simulink model "NMG_DMPC_Final"  (R2024b)
settings: Solver=VariableStepAuto  StartTime=0.0  StopTime=100  RelTol=1e-3
libraries: spspowerguiLib x1
settings Model: Creator=hp  LastModifiedBy=Ekko
settings SolverCC: AlgebraicLoopSolver=TrustRegion
settings DataIOCC: ReturnWorkspaceOutputs=off
settings DebuggingCC: UnconnectedInputMsg=warning  UnconnectedOutputMsg=warning  UnconnectedLineMsg=warning  ArithmeticOperatorsInVariantConditions=warning
settings ModelReferenceCC: EnableRefExpFcnMdlSchedulingChecks=on
settings SFSimCC: CustomCodeUndefinedFunction=UseInterfaceOnly
settings RTWCC: GPUComputeCapability=3.5

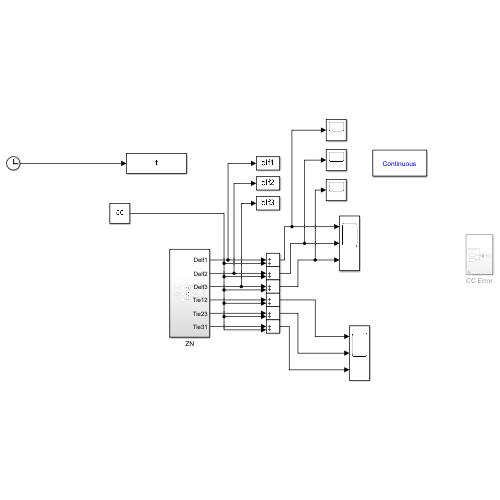
[thumbnail: Simulink's stored preview of the top-level diagram]
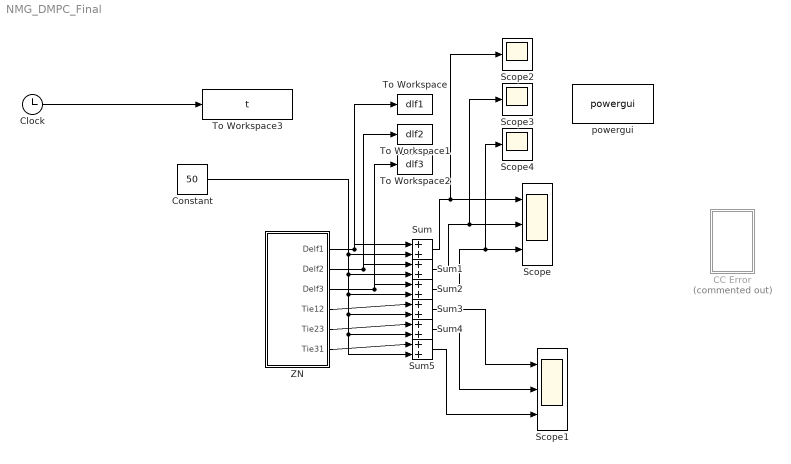
== system NMG_DMPC_Final ==
  CC Error : Subsystem  Commented=on
  Clock : Clock
  Constant : Constant  Value=50
  Scope : Scope  NumInputPorts=3
  Scope1 : Scope  NumInputPorts=3
  Scope2 : Scope
  Scope3 : Scope
  Scope4 : Scope
  Sum{,1..5} (6 alike) : Sum  Inputs=|++
  To Workspace : ToWorkspace  VariableName=dlf1  SampleTime=-1
      settings: Save2DSignal=2-D array (concatenate along first dimension)
  To Workspace1 : ToWorkspace  VariableName=dlf2  SampleTime=-1
      settings: Save2DSignal=2-D array (concatenate along first dimension)
  To Workspace2 : ToWorkspace  VariableName=dlf3  SampleTime=-1
      settings: Save2DSignal=2-D array (concatenate along first dimension)
  To Workspace3 : ToWorkspace  VariableName=t  SampleTime=-1
      settings: Save2DSignal=2-D array (concatenate along first dimension)
  ZN : Subsystem
  powergui : spspowerguiLib/powergui  Priority=1  SimulationMode=Continuous  SampleTime=50e-6  frequency=60  Iterations=50  frequencyindice=60  Pbase=100e6  ErrMax=1e-4  UnitsV=kV  UnitsW=MW  buscounter=0  FunctionMessages=off  echomessages=off  EnableUseOfTLC=off  CurrentSourceSwitches=off  DisableSnubberDevices=off  DisableRonSwitches=off  DisableVfSwitches=off  DisplayEquations=off  AutomaticDiscreteSolvers=off  SolverType=Tustin/Backward Euler (TBE)  Interpol=off  ExternalGateDelay=off  methode=off  Ts=100  x0status=blocks  SPID=on  SwTol=0  HookPort=off  NonlinearTolerance=1e-4  nMaxIteration=100  ContinueOnMaxIteration=off  RestoreLinks=warning  ResistiveCurrentMeasurement=off  Frange=[0:2:500]  Ylog=off  Xlog=on  ShowGrid=off  save=off  variable=ZData  structure=0  ZoomFFT=off  StartTime=0.0  cycles=1  DisplayStyle=1  fundamental=60  FreqAxis=off  MaxFrequency=1000  frequencyindicesteady=1  RmsSteady=1  display=off
  wires:
  ZN/1(Delf1) -> Sum/1, To Workspace/1
  Sum/1 -> Scope/1, Scope2/1
  Constant/1 -> Sum1/2, Sum3/2, Sum4/2, Sum5/2, Sum2/2, Sum/2
  ZN/2(Delf2) -> Sum1/1, To Workspace1/1
  ZN/3(Delf3) -> To Workspace2/1, Sum2/1
  Sum1/1 -> Scope3/1, Scope/2
  Sum2/1 -> Scope4/1, Scope/3
  ZN/4(Tie12) -> Sum3/1
  ZN/5(Tie23) -> Sum4/1
  ZN/6(Tie31) -> Sum5/1
  Sum3/1 -> Scope1/1
  Sum4/1 -> Scope1/2
  Sum5/1 -> Scope1/3
  Clock/1 -> To Workspace3/1

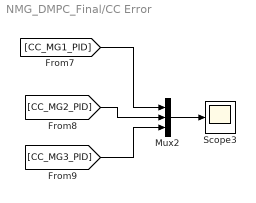
== system NMG_DMPC_Final/CC Error ==
  Mux2 : Mux  Inputs=3
  Scope3 : Scope
  wires:
  [CC_MG3_PID] -> Mux2/3
  Mux2/1 -> Scope3/1
  [CC_MG1_PID] -> Mux2/1
  [CC_MG2_PID] -> Mux2/2

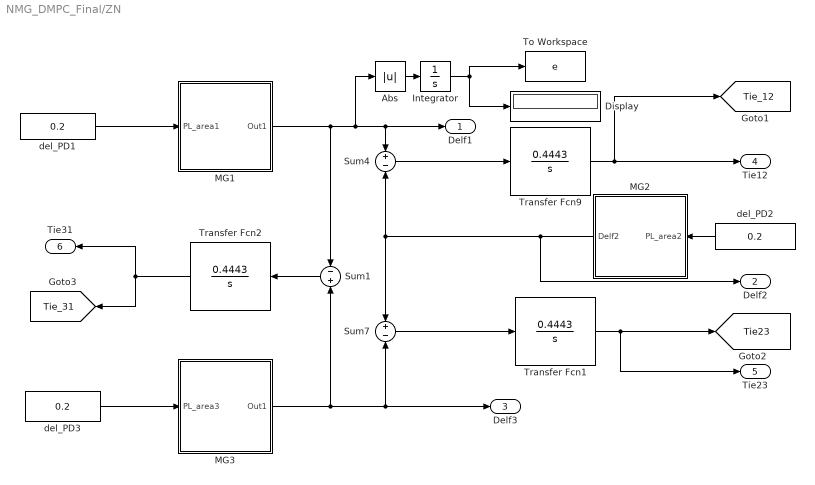
== system NMG_DMPC_Final/ZN ==
  Abs : Abs  SaturateOnIntegerOverflow=off
  Display : Display
  Integrator : Integrator
  MG1 : Subsystem
  MG2 : Subsystem
  MG3 : Subsystem
  Sum1 : Sum  Inputs=-+
  Sum4 : Sum  Inputs=+-
  Sum7 : Sum  Inputs=+-
  To Workspace : ToWorkspace  VariableName=e  SaveFormat=Timeseries  SampleTime=-1
  Transfer Fcn1 : TransferFcn  Numerator=[0.4443]  Denominator=[1 0]
  Transfer Fcn2 : TransferFcn  Numerator=[0.4443]  Denominator=[1 0]
  Transfer Fcn9 : TransferFcn  Numerator=[0.4443]  Denominator=[1 0]
  del_PD1 : Constant  Value=0.2
  del_PD2 : Constant  Value=0.2
  del_PD3 : Constant  Value=0.2
  Delf1 : Outport  VectorParamsAs1DForOutWhenUnconnected=off
  Delf2 : Outport  Port=2  VectorParamsAs1DForOutWhenUnconnected=off
  Delf3 : Outport  Port=3  VectorParamsAs1DForOutWhenUnconnected=off
  Tie12 : Outport  Port=4  VectorParamsAs1DForOutWhenUnconnected=off
  Tie23 : Outport  Port=5  VectorParamsAs1DForOutWhenUnconnected=off
  Tie31 : Outport  Port=6  VectorParamsAs1DForOutWhenUnconnected=off
  tag scope: Tie23=global, Tie_12=global, Tie_31=global
  wires:
  MG3/1(Out1) -> Delf3/1, Sum7/2, Sum1/2
  Sum7/1 -> Transfer Fcn1/1
  Sum4/1 -> Transfer Fcn9/1
  Transfer Fcn1/1 -> Tie23/1, [Tie23]
  Transfer Fcn9/1 -> [Tie_12], Tie12/1
  Sum1/1 -> Transfer Fcn2/1
  Transfer Fcn2/1 -> Tie31/1, [Tie_31]
  Integrator/1 -> Display/1, To Workspace/1
  MG1/1(Out1) -> Sum1/1, Abs/1, Sum4/1, Delf1/1
  Abs/1 -> Integrator/1
  del_PD2/1 -> MG2/1(PL_area2)
  del_PD3/1 -> MG3/1(PL_area3)
  del_PD1/1 -> MG1/1(PL_area1)
  MG2/1(Delf2) -> Sum7/1, Sum4/2, Delf2/1

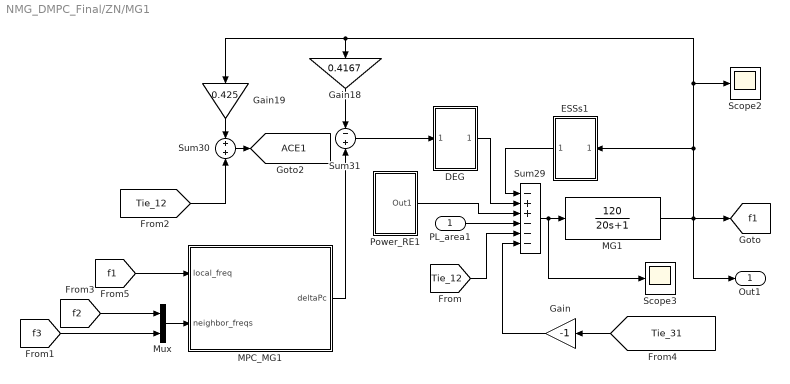
== system NMG_DMPC_Final/ZN/MG1 ==
  PL_area1 : Inport
  DEG : Subsystem
  ESSs1 : Subsystem
  Gain : Gain  Gain=-1
  Gain18 : Gain  Gain=0.4167
  Gain19 : Gain  Gain=0.425
  MG1 : TransferFcn  Numerator=[120]  Denominator=[20 1]
  MPC_MG1 : MATLAB Function  TreatAsAtomicUnit=on
  Mux : Mux  Inputs=2
  Power_RE1 : Subsystem
  Scope2 : Scope
  Scope3 : Scope
  Sum29 : Sum  Inputs=-++---
  Sum30 : Sum
  Sum31 : Sum  Inputs=-+
  Out1 : Outport  VectorParamsAs1DForOutWhenUnconnected=off
  tag scope: ACE1=global, f1=global
  wires:
  ESSs1/1(Out1) -> Sum29/1
  [Tie_12] -> Sum29/5
  MG1/1 -> [f1], Out1/1, ESSs1/1(In1), Scope2/1, Gain19/1, Gain18/1
  Sum29/1 -> Scope3/1, MG1/1
  Gain18/1 -> Sum31/1
  [Tie_12] -> Sum30/2
  MPC_MG1/1(deltaPc) -> Sum31/2
  Gain19/1 -> Sum30/1
  PL_area1/1 -> Sum29/4
  DEG/1(Out1) -> Sum29/2
  Power_RE1/1(Out1) -> Sum29/3
  Sum31/1 -> DEG/1(In1)
  [Tie_31] -> Gain/1
  Gain/1 -> Sum29/6
  Sum30/1 -> [ACE1]
  Mux/1 -> MPC_MG1/2(neighbor_freqs)
  [f2] -> Mux/1
  [f3] -> Mux/2
  [f1] -> MPC_MG1/1(local_freq)

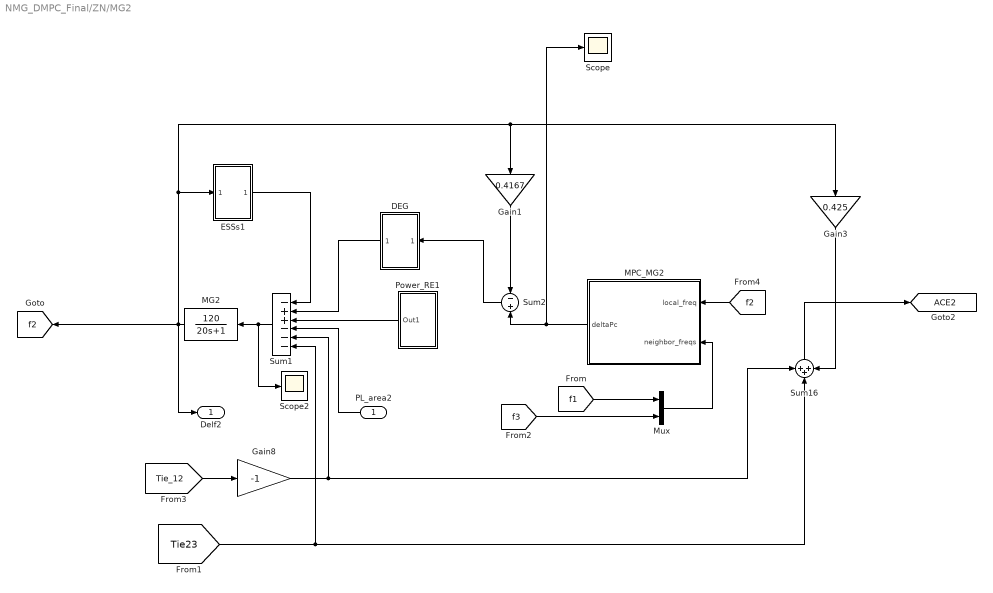
== system NMG_DMPC_Final/ZN/MG2 ==
  PL_area2 : Inport
  DEG : Subsystem
  ESSs1 : Subsystem
  Gain1 : Gain  Gain=0.4167
  Gain3 : Gain  Gain=0.425
  Gain8 : Gain  Gain=-1
  MG2 : TransferFcn  Numerator=[120]  Denominator=[20 1]
  MPC_MG2 : MATLAB Function  TreatAsAtomicUnit=on
  Mux : Mux  Inputs=2
  Power_RE1 : Subsystem
  Scope : Scope
  Scope2 : Scope
  Sum1 : Sum  Inputs=-++---
  Sum16 : Sum  Inputs=+++
  Sum2 : Sum  Inputs=-+
  Delf2 : Outport  VectorParamsAs1DForOutWhenUnconnected=off
  tag scope: ACE2=global, f2=global
  wires:
  [Tie23] -> Sum1/6, Sum16/2
  [Tie_12] -> Gain8/1
  MG2/1 -> ESSs1/1(In1), Gain1/1, Gain3/1, [f2], Delf2/1
  Gain8/1 -> Sum1/5, Sum16/1
  PL_area2/1 -> Sum1/4
  Gain1/1 -> Sum2/1
  MPC_MG2/1(deltaPc) -> Scope/1, Sum2/2
  Sum1/1 -> Scope2/1, MG2/1
  ESSs1/1(Out1) -> Sum1/1
  Gain3/1 -> Sum16/3
  DEG/1(Out1) -> Sum1/2
  Power_RE1/1(Out1) -> Sum1/3
  Sum2/1 -> DEG/1(In1)
  Sum16/1 -> [ACE2]
  Mux/1 -> MPC_MG2/2(neighbor_freqs)
  [f1] -> Mux/1
  [f3] -> Mux/2
  [f2] -> MPC_MG2/1(local_freq)

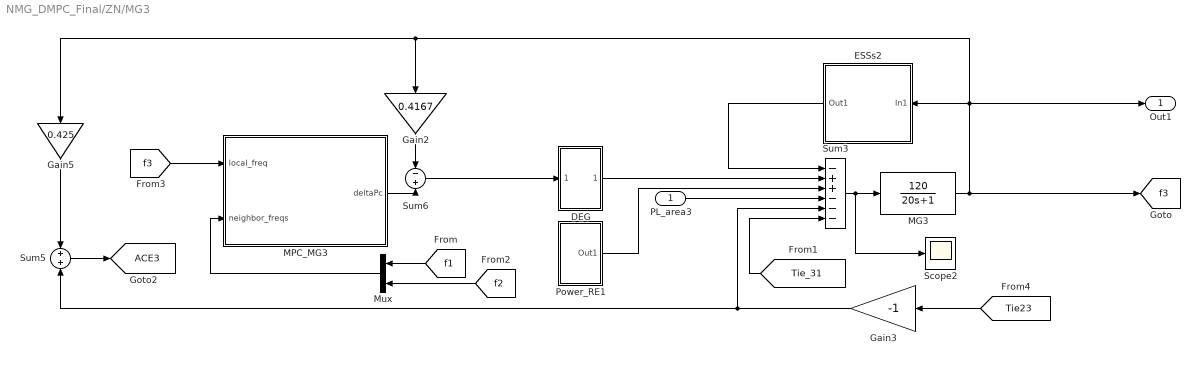
== system NMG_DMPC_Final/ZN/MG3 ==
  PL_area3 : Inport
  DEG : Subsystem
  ESSs2 : Subsystem
  Gain2 : Gain  Gain=0.4167
  Gain3 : Gain  Gain=-1
  Gain5 : Gain  Gain=0.425
  MG3 : TransferFcn  Numerator=[120]  Denominator=[20 1]
  MPC_MG3 : MATLAB Function  TreatAsAtomicUnit=on
  Mux : Mux  Inputs=2
  Power_RE1 : Subsystem
  Scope2 : Scope
  Sum3 : Sum  Inputs=-++---
  Sum5 : Sum
  Sum6 : Sum  Inputs=-+
  Out1 : Outport  VectorParamsAs1DForOutWhenUnconnected=off
  tag scope: ACE3=global, f3=global
  wires:
  MPC_MG3/1(deltaPc) -> Sum6/2
  Gain3/1 -> Sum3/5, Sum5/2
  MG3/1 -> [f3], Gain5/1, Gain2/1, Out1/1, ESSs2/1(In1)
  [Tie23] -> Gain3/1
  ESSs2/1(Out1) -> Sum3/1
  Gain2/1 -> Sum6/1
  Sum3/1 -> Scope2/1, MG3/1
  PL_area3/1 -> Sum3/4
  Power_RE1/1(Out1) -> Sum3/3
  Gain5/1 -> Sum5/1
  DEG/1(Out1) -> Sum3/2
  Sum6/1 -> DEG/1(In1)
  [Tie_31] -> Sum3/6
  Sum5/1 -> [ACE3]
  Mux/1 -> MPC_MG3/2(neighbor_freqs)
  [f2] -> Mux/2
  [f1] -> Mux/1
  [f3] -> MPC_MG3/1(local_freq)

== system NMG_DMPC_Final/ZN/MG1/DEG ==
  In1 : Inport
  Transfer Fcn15 : TransferFcn  Denominator=[1 1]
  Transfer Fcn22 : TransferFcn  Denominator=[2 1]
  Out1 : Outport  VectorParamsAs1DForOutWhenUnconnected=off
  wires:
  Transfer Fcn22/1 -> Transfer Fcn15/1
  In1/1 -> Transfer Fcn22/1
  Transfer Fcn15/1 -> Out1/1

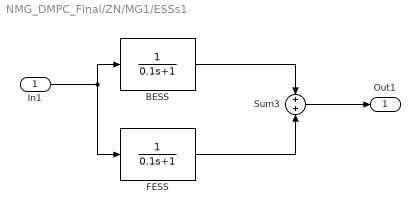
== system NMG_DMPC_Final/ZN/MG1/ESSs1 ==
  In1 : Inport
  BESS : TransferFcn  Denominator=[0.1 1]
  FESS : TransferFcn  Denominator=[0.1 1]
  Sum3 : Sum
  Out1 : Outport  VectorParamsAs1DForOutWhenUnconnected=off
  wires:
  In1/1 -> FESS/1, BESS/1
  Sum3/1 -> Out1/1
  FESS/1 -> Sum3/2
  BESS/1 -> Sum3/1

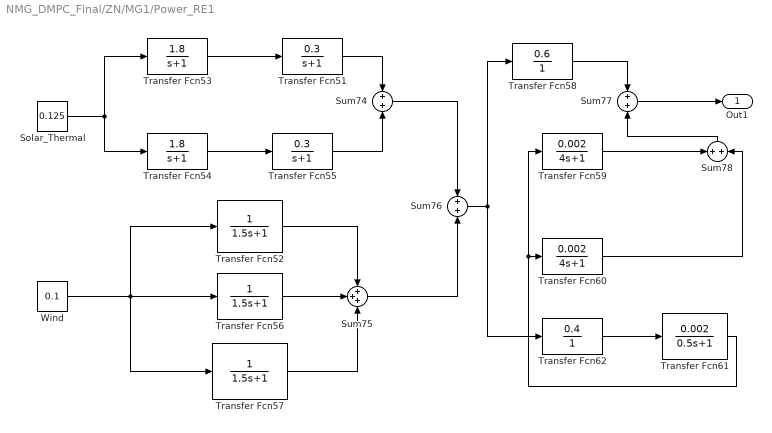
== system NMG_DMPC_Final/ZN/MG1/Power_RE1 ==
  Solar_Thermal : Constant  Value=0.125
  Sum{74,76..78} (4 alike) : Sum
  Sum75 : Sum  Inputs=+++
  Transfer Fcn51 : TransferFcn  Numerator=[0.3]  Denominator=[1 1]
  Transfer Fcn52 : TransferFcn  Denominator=[1.5 1]
  Transfer Fcn53 : TransferFcn  Numerator=[1.8]  Denominator=[1 1]
  Transfer Fcn54 : TransferFcn  Numerator=[1.8]  Denominator=[1 1]
  Transfer Fcn55 : TransferFcn  Numerator=[0.3]  Denominator=[1 1]
  Transfer Fcn56 : TransferFcn  Denominator=[1.5 1]
  Transfer Fcn57 : TransferFcn  Denominator=[1.5 1]
  Transfer Fcn58 : TransferFcn  Numerator=[0.6]  Denominator=[1]
  Transfer Fcn59 : TransferFcn  Numerator=[0.002]  Denominator=[4 1]
  Transfer Fcn60 : TransferFcn  Numerator=[0.002]  Denominator=[4 1]
  Transfer Fcn61 : TransferFcn  Numerator=[0.002]  Denominator=[0.5 1]
  Transfer Fcn62 : TransferFcn  Numerator=[0.4]  Denominator=[1]
  Wind : Constant  Value=0.1
  Out1 : Outport  VectorParamsAs1DForOutWhenUnconnected=off
  wires:
  Transfer Fcn52/1 -> Sum75/1
  Transfer Fcn53/1 -> Transfer Fcn51/1
  Solar_Thermal/1 -> Transfer Fcn53/1, Transfer Fcn54/1
  Transfer Fcn51/1 -> Sum74/1
  Transfer Fcn60/1 -> Sum78/2
  Transfer Fcn56/1 -> Sum75/2
  Wind/1 -> Transfer Fcn57/1, Transfer Fcn56/1, Transfer Fcn52/1
  Transfer Fcn57/1 -> Sum75/3
  Transfer Fcn58/1 -> Sum77/1
  Sum75/1 -> Sum76/2
  Sum78/1 -> Sum77/2
  Sum74/1 -> Sum76/1
  Transfer Fcn54/1 -> Transfer Fcn55/1
  Transfer Fcn55/1 -> Sum74/2
  Transfer Fcn61/1 -> Transfer Fcn60/1, Transfer Fcn59/1
  Transfer Fcn59/1 -> Sum78/1
  Sum76/1 -> Transfer Fcn58/1, Transfer Fcn62/1
  Transfer Fcn62/1 -> Transfer Fcn61/1
  Sum77/1 -> Out1/1

== system NMG_DMPC_Final/ZN/MG2/DEG ==
  In1 : Inport
  Transfer Fcn15 : TransferFcn  Denominator=[1 1]
  Transfer Fcn22 : TransferFcn  Denominator=[2 1]
  Out1 : Outport  VectorParamsAs1DForOutWhenUnconnected=off
  wires:
  Transfer Fcn22/1 -> Transfer Fcn15/1
  In1/1 -> Transfer Fcn22/1
  Transfer Fcn15/1 -> Out1/1

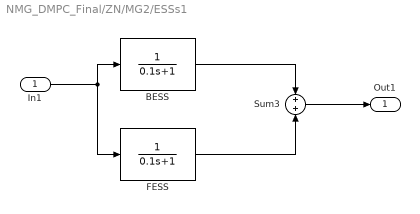
== system NMG_DMPC_Final/ZN/MG2/ESSs1 ==
  In1 : Inport
  BESS : TransferFcn  Denominator=[0.1 1]
  FESS : TransferFcn  Denominator=[0.1 1]
  Sum3 : Sum
  Out1 : Outport  VectorParamsAs1DForOutWhenUnconnected=off
  wires:
  In1/1 -> FESS/1, BESS/1
  Sum3/1 -> Out1/1
  FESS/1 -> Sum3/2
  BESS/1 -> Sum3/1

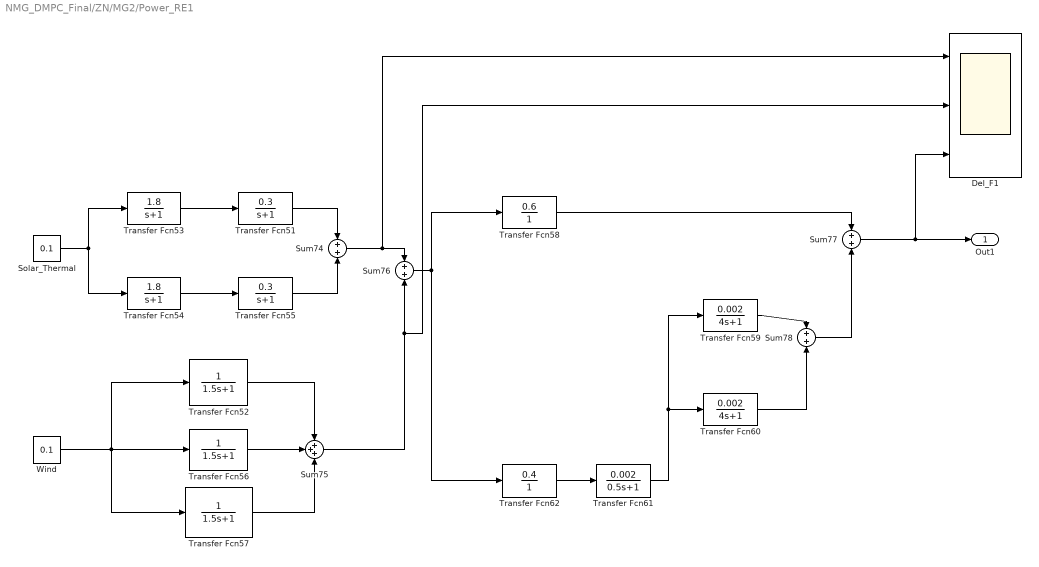
== system NMG_DMPC_Final/ZN/MG2/Power_RE1 ==
  Del_F1 : Scope  NumInputPorts=3
  Solar_Thermal : Constant  Value=0.1
  Sum{74,76..78} (4 alike) : Sum
  Sum75 : Sum  Inputs=+++
  Transfer Fcn51 : TransferFcn  Numerator=[0.3]  Denominator=[1 1]
  Transfer Fcn52 : TransferFcn  Denominator=[1.5 1]
  Transfer Fcn53 : TransferFcn  Numerator=[1.8]  Denominator=[1 1]
  Transfer Fcn54 : TransferFcn  Numerator=[1.8]  Denominator=[1 1]
  Transfer Fcn55 : TransferFcn  Numerator=[0.3]  Denominator=[1 1]
  Transfer Fcn56 : TransferFcn  Denominator=[1.5 1]
  Transfer Fcn57 : TransferFcn  Denominator=[1.5 1]
  Transfer Fcn58 : TransferFcn  Numerator=[0.6]  Denominator=[1]
  Transfer Fcn59 : TransferFcn  Numerator=[0.002]  Denominator=[4 1]
  Transfer Fcn60 : TransferFcn  Numerator=[0.002]  Denominator=[4 1]
  Transfer Fcn61 : TransferFcn  Numerator=[0.002]  Denominator=[0.5 1]
  Transfer Fcn62 : TransferFcn  Numerator=[0.4]  Denominator=[1]
  Wind : Constant  Value=0.1
  Out1 : Outport  VectorParamsAs1DForOutWhenUnconnected=off
  wires:
  Transfer Fcn52/1 -> Sum75/1
  Transfer Fcn53/1 -> Transfer Fcn51/1
  Solar_Thermal/1 -> Transfer Fcn54/1, Transfer Fcn53/1
  Transfer Fcn51/1 -> Sum74/1
  Transfer Fcn60/1 -> Sum78/2
  Transfer Fcn56/1 -> Sum75/2
  Wind/1 -> Transfer Fcn52/1, Transfer Fcn56/1, Transfer Fcn57/1
  Transfer Fcn57/1 -> Sum75/3
  Transfer Fcn58/1 -> Sum77/1
  Sum75/1 -> Del_F1/2, Sum76/2
  Sum78/1 -> Sum77/2
  Sum74/1 -> Del_F1/1, Sum76/1
  Transfer Fcn54/1 -> Transfer Fcn55/1
  Transfer Fcn55/1 -> Sum74/2
  Transfer Fcn61/1 -> Transfer Fcn60/1, Transfer Fcn59/1
  Transfer Fcn59/1 -> Sum78/1
  Sum76/1 -> Transfer Fcn62/1, Transfer Fcn58/1
  Transfer Fcn62/1 -> Transfer Fcn61/1
  Sum77/1 -> Del_F1/3, Out1/1

== system NMG_DMPC_Final/ZN/MG3/DEG ==
  In1 : Inport
  Transfer Fcn15 : TransferFcn  Denominator=[1 1]
  Transfer Fcn22 : TransferFcn  Denominator=[2 1]
  Out1 : Outport  VectorParamsAs1DForOutWhenUnconnected=off
  wires:
  Transfer Fcn22/1 -> Transfer Fcn15/1
  In1/1 -> Transfer Fcn22/1
  Transfer Fcn15/1 -> Out1/1

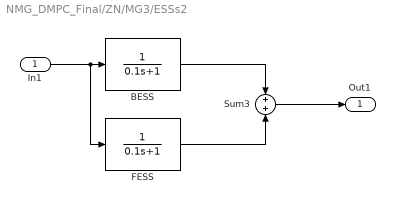
== system NMG_DMPC_Final/ZN/MG3/ESSs2 ==
  In1 : Inport
  BESS : TransferFcn  Denominator=[0.1 1]
  FESS : TransferFcn  Denominator=[0.1 1]
  Sum3 : Sum
  Out1 : Outport  VectorParamsAs1DForOutWhenUnconnected=off
  wires:
  BESS/1 -> Sum3/1
  FESS/1 -> Sum3/2
  In1/1 -> FESS/1, BESS/1
  Sum3/1 -> Out1/1

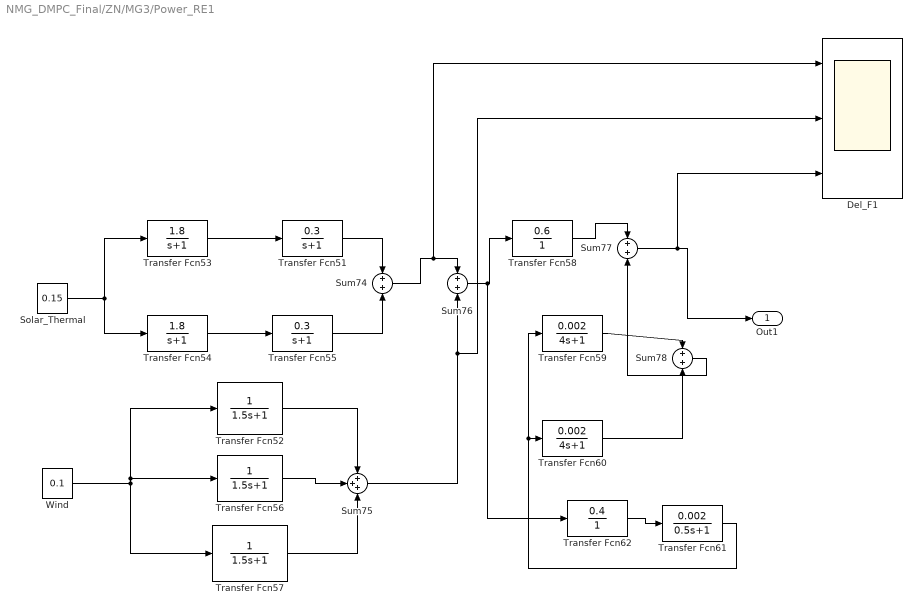
== system NMG_DMPC_Final/ZN/MG3/Power_RE1 ==
  Del_F1 : Scope  NumInputPorts=3
  Solar_Thermal : Constant  Value=0.15
  Sum{74,76..78} (4 alike) : Sum
  Sum75 : Sum  Inputs=+++
  Transfer Fcn51 : TransferFcn  Numerator=[0.3]  Denominator=[1 1]
  Transfer Fcn52 : TransferFcn  Denominator=[1.5 1]
  Transfer Fcn53 : TransferFcn  Numerator=[1.8]  Denominator=[1 1]
  Transfer Fcn54 : TransferFcn  Numerator=[1.8]  Denominator=[1 1]
  Transfer Fcn55 : TransferFcn  Numerator=[0.3]  Denominator=[1 1]
  Transfer Fcn56 : TransferFcn  Denominator=[1.5 1]
  Transfer Fcn57 : TransferFcn  Denominator=[1.5 1]
  Transfer Fcn58 : TransferFcn  Numerator=[0.6]  Denominator=[1]
  Transfer Fcn59 : TransferFcn  Numerator=[0.002]  Denominator=[4 1]
  Transfer Fcn60 : TransferFcn  Numerator=[0.002]  Denominator=[4 1]
  Transfer Fcn61 : TransferFcn  Numerator=[0.002]  Denominator=[0.5 1]
  Transfer Fcn62 : TransferFcn  Numerator=[0.4]  Denominator=[1]
  Wind : Constant  Value=0.1
  Out1 : Outport  VectorParamsAs1DForOutWhenUnconnected=off
  wires:
  Transfer Fcn52/1 -> Sum75/1
  Transfer Fcn53/1 -> Transfer Fcn51/1
  Solar_Thermal/1 -> Transfer Fcn53/1, Transfer Fcn54/1
  Transfer Fcn51/1 -> Sum74/1
  Transfer Fcn60/1 -> Sum78/2
  Transfer Fcn56/1 -> Sum75/2
  Wind/1 -> Transfer Fcn56/1, Transfer Fcn52/1, Transfer Fcn57/1
  Transfer Fcn57/1 -> Sum75/3
  Transfer Fcn58/1 -> Sum77/1
  Sum75/1 -> Del_F1/2, Sum76/2
  Sum78/1 -> Sum77/2
  Sum74/1 -> Del_F1/1, Sum76/1
  Transfer Fcn54/1 -> Transfer Fcn55/1
  Transfer Fcn55/1 -> Sum74/2
  Transfer Fcn61/1 -> Transfer Fcn60/1, Transfer Fcn59/1
  Transfer Fcn59/1 -> Sum78/1
  Sum76/1 -> Transfer Fcn62/1, Transfer Fcn58/1
  Transfer Fcn62/1 -> Transfer Fcn61/1
  Sum77/1 -> Del_F1/3, Out1/1

== matlab function NMG_DMPC_Final/ZN/MG1/MPC_MG1 ==
  settings: updateMethod=DISCRETE
  data: local_freq input; deltaPc output; neighbor_freqs input
function deltaPc = MPC_MG1(local_freq, neighbor_freqs)
    % System Parameters
    Ts = 0.01;          % Fixed sampling time (seconds)
    R_droop = 0.41667;  % Droop constant
    T12 = 0.4443;       % Tie-line coefficient MG1-MG2
    T31 = 0.4443;       % Tie-line coefficient MG3-MG1
    
    % MPC Design Parameters - Ultimate stability configuration
    Np = 20;        % Very long prediction horizon for maximum stability
    Nc = 5;         % Minimal control horizon for extremely smooth action
    
    % State-Space Matrices
    % States: [DEG(2) Solar(4) Wind(3) RE_Out(4) ESS(2) PS(3)]
    A = zeros(18, 18);  % Initialize with zeros for clarity
    
    % Fill in the A matrix blocks (keep your existing A matrix setup)
    % DEG dynamics (states 1-2)
    A(1:2, 1:2) = [-1/2, 0;
                    1,  -1];
    
    % Solar-Thermal (states 3-6)
    A(3:6, 3:6) = [-1,   1.8,   0,    0;
                    0,    -1,    0,    0;
                    0,     0,   -1,   0.3;
                    0,     0,    0,   -1];
                    
    % Wind (states 7-9)
    A(7:9, 7:9) = [-2/3,  0,    0;
                     0,   -2/3,  0;
                     0,    0,   -2/3];
                     
    % RE Output Stage (states 10-13)
    A(10, 3:9) = [1, 0, 1, 0, 1, 1, 1];  % Connections from Solar and Wind
    A(10:13, 10:13) = [-1/4,  0,    0,    0;
                        0,   -1/4,   0,    0;
                        0,    0.6,   0,    0;
                        0,     0,    0,   -2];
                        
    % ESS (states 14-15)
    A(14:15, 14:15) = [-10,  0;
                         0, -10];
                         
    % Power System & Tie-lines (states 16-18)
    A(16, [1,10:15]) = [120/20, 120/20, 120/20, 120/20, 120/20, 120/20, 120/20];  % Effects on frequency
    A(16:18, 16:18) = [-1/20,  0,    0;
                        T12,    0,    0;  % Tie-line to MG2
                        T31,    0,    0];  % Tie-line to MG3
    
    % Input matrix B
    B = zeros(18, 1);
    B(1) = 1/2;  % Control input only affects DEG first state
    
    % Output matrix C - only measure frequency for control
    C = zeros(1, 18);
    C(16) = 1;  % Measure frequency state
    
    % Augmented System
    A_aug = [A, zeros(18,1);
             C, 0];
    B_aug = [B; 0];
    C_aug = [C, 0];
    
    % Discrete-time conversion
    Ad = eye(19) + Ts*A_aug;
    Bd = Ts*B_aug;
    Cd = C_aug;
    
    % Persistent variables with enhanced filtering
    persistent x_est u_prev integral_error avg_error filter_count
    persistent y_hist error_trend deltaPc_hist prev_solution
    persistent y_filtered_prev deltaPc_final_prev
    if isempty(x_est)
        x_est = zeros(19, 1);
        u_prev = 0;
        integral_error = 0;
        avg_error = 0;
        filter_count = 0;
        y_hist = zeros(8, 1);
        error_trend = zeros(5, 1);
        deltaPc_hist = zeros(3, 1);
        prev_solution = zeros(Nc, 1);
        y_filtered_prev = 0;
        deltaPc_final_prev = 0;
    end
    
    % Extract frequency information from neighbors
    freq_MG2 = neighbor_freqs(1);
    freq_MG3 = neighbor_freqs(2);
    
    % Distributed Control Based on Laplacian Matrix
    % For MG1 (Leader): Use direct reference tracking + neighboring information
    reference = 50.0;  % Reference frequency
    graph_gain = 0.2;  % Gain for graph-based control
    
    % Calculate distributed control error using graph theory
    % Based on local error + weighted neighbor errors
    laplacian_error = 2*local_freq - freq_MG2 - freq_MG3;
    reference_error = local_freq - reference;
    
    % Combined error (leader node has direct access to reference)
    dist_error = reference_error + graph_gain*laplacian_error;
    
    % Enhanced measurement filtering with longer history and stronger filtering
    y_hist = [dist_error; y_hist(1:end-1)];
    
    % Two-stage filtering for maximum noise rejection
    % First stage: weighted moving average
    weights = [0.25, 0.2, 0.15, 0.1, 0.1, 0.08, 0.07, 0.05];
    weights = weights(1:min(length(weights), length(y_hist)));
    weights = weights / sum(weights);
    y_filtered_stage1 = y_hist' * weights';
    
    % Second stage: low-pass filter
    if isempty(y_filtered_prev)
        y_filtered_prev = y_filtered_stage1;
    end
    y_filtered = 0.8*y_filtered_prev + 0.2*y_filtered_stage1;
    y_filtered_prev = y_filtered;
    
    % Ultra-conservative integral action with wider dead zone
    error_signal = y_filtered;
    
    % Expanded dead zone with extremely slow integration
    if abs(error_signal) > 0.01
        integral_error = 0.99*integral_error + 0.01*Ts*error_signal*0.05;
    else
        % Inside dead zone - practically frozen integration
        integral_error = 0.9995*integral_error + 0.0005*Ts*error_signal*0.01;
    end
    
    % Moving average error for steady-state offset detection
    avg_error = 0.95*avg_error + 0.05*error_signal;
    filter_count = filter_count + 1;
    
    % State estimation with improved observer gain
    y_meas = y_filtered;
    x_est = Ad*x_est + Bd*u_prev;
    
    % Slightly increased observer gain for better tracking
    L = [0.08*ones(18,1); 0.12];
    x_est = x_est + L*(y_meas - Cd*x_est);
    x_est(19) = integral_error;
    
    % Prediction matrices
    [F, Phi] = getPredictionMatrices(Ad, Bd, Cd, Np, Nc);
    
    % Cost function weights - Critically over-damped response design
    % Extremely flat weight distribution for maximum smoothness
    %q_weights = exp(linspace(0, 0.2, Np));  % Very gradual weight increase
    Q = diag(500 * exp(linspace(0, 0.5, Np)));  % Sharper tracking
    
    % Ultra-high penalty on control moves to eliminate any oscillatory behavior
    R = diag(0.8 * ones(Nc,1));                 % Reduced control penalty
    
    % Reference trajectory - Targeting zero error
    r = zeros(Np,1);
    
    % Constraints - Extremely tight rate constraints for absolute stability
    du_max = 0.01;      % Minimal rate of change allowed
    u_max = 0.13;
    u_min = -0.13;
    
    % QP matrices
    [H, f] = getQPMatrices(F, Phi, Q, R, r, x_est);
    [A_ineq, b_ineq] = getConstraintMatrices(Nc, u_max, u_min, du_max, u_prev);
    
    % Initial guess - Use previous solution as starting point if available
    x0 = prev_solution;
    
    % Solve QP problem with improved options
    options = optimoptions('quadprog', 'Display', 'off', 'Algorithm', 'active-set', ...
                          'MaxIterations', 100);
    du = quadprog(H, f, A_ineq, b_ineq, [], [], [], [], x0, options);
    
    % Store solution for next iteration
    if ~isempty(du)
        prev_solution = du;
        delta_u = du(1);
    else
        delta_u = 0;
    end
    
    % Add anti-windup to prevent integral windup
    if abs(u_prev) >= u_max - 0.01
        integral_error = 0.9 * integral_error; % Reduce integral action when near constraints
    end
    
    % Maximum damping factor with triple-stage filtering
    % First stage - exponential smoothing with heavy bias toward previous value
    deltaPc_stage1 = 0.85*u_prev + 0.15*delta_u;
    
    % Second stage - moving average filter
    deltaPc_hist = [deltaPc_stage1; deltaPc_hist(1:end-1)];
    if all(deltaPc_hist == 0)
        deltaPc_hist = zeros(3, 1) + deltaPc_stage1;
    end
    deltaPc_stage2 = 0.7*deltaPc_hist(1) + 0.2*deltaPc_hist(2) + 0.1*deltaPc_hist(3);
    
    % Third stage - additional low-pass filter
    if isempty(deltaPc_final_prev)
        deltaPc_final_prev = deltaPc_stage2;
    end
    deltaPc = 0.9*deltaPc_final_prev + 0.1*deltaPc_stage2;
    deltaPc_final_prev = deltaPc;
    
    % Update persistent variables
    u_prev = deltaPc;
    
    return;
end

function [F, Phi] = getPredictionMatrices(A, B, C, Np, Nc)
    % Keep your existing function implementation
    [ny, nx] = size(C);
    F = zeros(Np, nx);
    Phi = zeros(Np, Nc);
    
    % Build F matrix
    for i = 1:Np
        F(i,:) = C * A^i;
    end
    
    % Build Phi matrix
    for i = 1:Np
        for j = 1:min(i,Nc)
            if i == j
                Phi(i,j) = C * B;
            else
                Phi(i,j) = C * A^(i-j) * B;
            end
        end
    end
end

function [H, f] = getQPMatrices(F, Phi, Q, R, r, x)
    % Keep your existing function implementation
    H = 2*(Phi'*Q*Phi + R);
    f = 2*Phi'*Q*(F*x - r);
end

function [A_ineq, b_ineq] = getConstraintMatrices(Nc, u_max, u_min, du_max, u_prev)
    % Keep your existing function implementation
    A_rate = [eye(Nc); -eye(Nc)];
    b_rate = [du_max*ones(Nc,1); du_max*ones(Nc,1)];
    
    A_input = tril(ones(Nc));
    A_amp = [A_input; -A_input];
    b_amp = [(u_max - u_prev)*ones(Nc,1); -(u_min - u_prev)*ones(Nc,1)];
    
    A_ineq = [A_rate; A_amp];
    b_ineq = [b_rate; b_amp];
end

== matlab function NMG_DMPC_Final/ZN/MG3/MPC_MG3 ==
  settings: updateMethod=DISCRETE
  data: local_freq input; deltaPc output; neighbor_freqs input
function deltaPc = MPC_MG3(local_freq, neighbor_freqs)
    % System Parameters
    Ts = 0.01;          % Fixed sampling time (seconds)
    R_droop = 0.41667;  % Droop constant
    T31 = 0.4443;       % Tie-line coefficient MG3-MG1
    T23 = 0.4443;       % Tie-line coefficient MG2-MG3
    
    % MPC Design Parameters - Ultimate stability configuration
    Np = 20;        % Very long prediction horizon for maximum stability
    Nc = 5;         % Minimal control horizon for extremely smooth action
    
    % State-Space Matrices
    % Keep your existing A matrix setup
    A = zeros(18, 18);  % Initialize with zeros for clarity
    
    % Fill in the A matrix blocks
    % DEG dynamics (states 1-2)
    A(1:2, 1:2) = [-1/2, 0;
                    1,  -1];
    
    % Solar-Thermal (states 3-6)
    A(3:6, 3:6) = [-1,   1.8,   0,    0;
                    0,    -1,    0,    0;
                    0,     0,   -1,   0.3;
                    0,     0,    0,   -1];
                    
    % Wind (states 7-9)
    A(7:9, 7:9) = [-2/3,  0,    0;
                     0,   -2/3,  0;
                     0,    0,   -2/3];
                     
    % RE Output Stage (states 10-13)
    A(10, 3:9) = [1, 0, 1, 0, 1, 1, 1];  % Connections from Solar and Wind
    A(10:13, 10:13) = [-1/4,  0,    0,    0;
                        0,   -1/4,   0,    0;
                        0,    0.6,   0,    0;
                        0,     0,    0,   -2];
                        
    % ESS (states 14-15)
    A(14:15, 14:15) = [-10,  0;
                         0, -10];
                         
    % Power System & Tie-lines (states 16-18)
    A(16, [1,10:15]) = [120/20, 120/20, 120/20, 120/20, 120/20, 120/20, 120/20];  % Effects on frequency
    A(16:18, 16:18) = [-1/20,  0,    0;
                        T31,    0,    0;  % Tie-line to MG1
                        T23,    0,    0];  % Tie-line to MG2
    
    % Input matrix B
    B = zeros(18, 1);
    B(1) = 1/2;  % Control input only affects DEG first state
    
    % Output matrix C - only measure frequency for control
    C = zeros(1, 18);
    C(16) = 1;  % Measure frequency state
    
    % Augmented System
    A_aug = [A, zeros(18,1);
             C, 0];
    B_aug = [B; 0];
    C_aug = [C, 0];
    
    % Discrete-time conversion
    Ad = eye(19) + Ts*A_aug;
    Bd = Ts*B_aug;
    Cd = C_aug;
    
    % Persistent variables with enhanced filtering
    persistent x_est u_prev integral_error avg_error filter_count
    persistent y_hist error_trend deltaPc_hist prev_solution
    persistent y_filtered_prev deltaPc_final_prev
    if isempty(x_est)
        x_est = zeros(19, 1);
        u_prev = 0;
        integral_error = 0;
        avg_error = 0;
        filter_count = 0;
        y_hist = zeros(8, 1);
        error_trend = zeros(5, 1);
        deltaPc_hist = zeros(3, 1);
        prev_solution = zeros(Nc, 1);
        y_filtered_prev = 0;
        deltaPc_final_prev = 0;
    end
    
    % Extract frequency information from neighbors
    freq_MG1 = neighbor_freqs(1);  % Leader frequency
    freq_MG2 = neighbor_freqs(2);
    
    % Distributed Control Based on Laplacian Matrix
    % For MG3 (Follower): Use neighboring information
    graph_gain = 0.2;  % Gain for graph-based control
    leader_gain = 0.5; % Higher gain for tracking the leader
    
    % Calculate distributed control error using graph theory
    % Based on local error + weighted neighbor errors
    laplacian_error = 2*local_freq - freq_MG1 - freq_MG2;
    leader_error = local_freq - freq_MG1;  % Track the leader
    
    % Combined error (follower node emphasizes tracking the leader)
    dist_error = leader_gain*leader_error + graph_gain*laplacian_error;
    
    % Enhanced measurement filtering with longer history and stronger filtering
    y_hist = [dist_error; y_hist(1:end-1)];
    
    % Two-stage filtering for maximum noise rejection
    % First stage: weighted moving average
    weights = [0.25, 0.2, 0.15, 0.1, 0.1, 0.08, 0.07, 0.05];
    weights = weights(1:min(length(weights), length(y_hist)));
    weights = weights / sum(weights);
    y_filtered_stage1 = y_hist' * weights';
    
    % Second stage: low-pass filter
    if isempty(y_filtered_prev)
        y_filtered_prev = y_filtered_stage1;
    end
    y_filtered = 0.8*y_filtered_prev + 0.2*y_filtered_stage1;
    y_filtered_prev = y_filtered;
    
    % Ultra-conservative integral action with wider dead zone
    error_signal = y_filtered;
    
    % Expanded dead zone with extremely slow integration
    if abs(error_signal) > 0.01
        integral_error = 0.99*integral_error + 0.01*Ts*error_signal*0.05;
    else
        % Inside dead zone - practically frozen integration
        integral_error = 0.9995*integral_error + 0.0005*Ts*error_signal*0.01;
    end
    
    % Moving average error for steady-state offset detection
    avg_error = 0.95*avg_error + 0.05*error_signal;
    filter_count = filter_count + 1;
    
    % State estimation with improved observer gain
    y_meas = y_filtered;
    x_est = Ad*x_est + Bd*u_prev;
    
    % Slightly increased observer gain for better tracking
    L = [0.08*ones(18,1); 0.12];
    x_est = x_est + L*(y_meas - Cd*x_est);
    x_est(19) = integral_error;
    
    % Prediction matrices
    [F, Phi] = getPredictionMatrices(Ad, Bd, Cd, Np, Nc);
    
    % Cost function weights - Critically over-damped response design
    % Extremely flat weight distribution for maximum smoothness
    %q_weights = exp(linspace(0, 0.2, Np));  % Very gradual weight increase
    Q = diag(500 * exp(linspace(0, 0.5, Np)));  % Sharper tracking
    
    % Ultra-high penalty on control moves to eliminate any oscillatory behavior
    R = diag(0.8 * ones(Nc,1));                 % Reduced control penalty
    
    % Reference trajectory - Targeting zero error
    r = zeros(Np,1);
    
    % Constraints - Extremely tight rate constraints for absolute stability
    du_max = 0.01;      % Minimal rate of change allowed
    u_max = 0.13;
    u_min = -0.13;
    % QP matrices
    [H, f] = getQPMatrices(F, Phi, Q, R, r, x_est);
    [A_ineq, b_ineq] = getConstraintMatrices(Nc, u_max, u_min, du_max, u_prev);
    
    % Initial guess - Use previous solution as starting point if available
    x0 = prev_solution;
    
    % Solve QP problem with improved options
    options = optimoptions('quadprog', 'Display', 'off', 'Algorithm', 'active-set', ...
                          'MaxIterations', 100);
    du = quadprog(H, f, A_ineq, b_ineq, [], [], [], [], x0, options);
    
    % Store solution for next iteration
    if ~isempty(du)
        prev_solution = du;
        delta_u = du(1);
    else
        delta_u = 0;
    end
    
    % Add anti-windup to prevent integral windup
    if abs(u_prev) >= u_max - 0.01
        integral_error = 0.9 * integral_error; % Reduce integral action when near constraints
    end
    
    % Maximum damping factor with triple-stage filtering
    % First stage - exponential smoothing with heavy bias toward previous value
    deltaPc_stage1 = 0.85*u_prev + 0.15*delta_u;
    
    % Second stage - moving average filter
    deltaPc_hist = [deltaPc_stage1; deltaPc_hist(1:end-1)];
    if all(deltaPc_hist == 0)
        deltaPc_hist = zeros(3, 1) + deltaPc_stage1;
    end
    deltaPc_stage2 = 0.7*deltaPc_hist(1) + 0.2*deltaPc_hist(2) + 0.1*deltaPc_hist(3);
    
    % Third stage - additional low-pass filter
    if isempty(deltaPc_final_prev)
        deltaPc_final_prev = deltaPc_stage2;
    end
    deltaPc = 0.9*deltaPc_final_prev + 0.1*deltaPc_stage2;
    deltaPc_final_prev = deltaPc;
    
    % Update persistent variables
    u_prev = deltaPc;
    
    return;
end

function [F, Phi] = getPredictionMatrices(A, B, C, Np, Nc)
    % Keep your existing function implementation
    [ny, nx] = size(C);
    F = zeros(Np, nx);
    Phi = zeros(Np, Nc);
    
    % Build F matrix
    for i = 1:Np
        F(i,:) = C * A^i;
    end
    
    % Build Phi matrix
    for i = 1:Np
        for j = 1:min(i,Nc)
            if i == j
                Phi(i,j) = C * B;
            else
                Phi(i,j) = C * A^(i-j) * B;
            end
        end
    end
end

function [H, f] = getQPMatrices(F, Phi, Q, R, r, x)
    % Keep your existing function implementation
    H = 2*(Phi'*Q*Phi + R);
    f = 2*Phi'*Q*(F*x - r);
end

function [A_ineq, b_ineq] = getConstraintMatrices(Nc, u_max, u_min, du_max, u_prev)
    % Keep your existing function implementation
    A_rate = [eye(Nc); -eye(Nc)];
    b_rate = [du_max*ones(Nc,1); du_max*ones(Nc,1)];
    
    A_input = tril(ones(Nc));
    A_amp = [A_input; -A_input];
    b_amp = [(u_max - u_prev)*ones(Nc,1); -(u_min - u_prev)*ones(Nc,1)];
    
    A_ineq = [A_rate; A_amp];
    b_ineq = [b_rate; b_amp];
end

== matlab function NMG_DMPC_Final/ZN/MG2/MPC_MG2 ==
  settings: updateMethod=DISCRETE
  data: local_freq input; deltaPc output; neighbor_freqs input
function deltaPc = MPC_MG2(local_freq, neighbor_freqs)
    % System Parameters
    Ts = 0.01;          % Fixed sampling time (seconds)
    R_droop = 0.41667;  % Droop constant
    T12 = 0.4443;       % Tie-line coefficient MG1-MG2
    T23 = 0.4443;       % Tie-line coefficient MG2-MG3
    
    % MPC Design Parameters - Ultimate stability configuration
    Np = 20;        % Very long prediction horizon for maximum stability
    Nc = 5;         % Minimal control horizon for extremely smooth action
    
    % State-Space Matrices
    % Keep your existing A matrix setup
    A = zeros(18, 18);  % Initialize with zeros for clarity
    
    % Fill in the A matrix blocks
    % DEG dynamics (states 1-2)
    A(1:2, 1:2) = [-1/2, 0;
                    1,  -1];
    
    % Solar-Thermal (states 3-6)
    A(3:6, 3:6) = [-1,   1.8,   0,    0;
                    0,    -1,    0,    0;
                    0,     0,   -1,   0.3;
                    0,     0,    0,   -1];
                    
    % Wind (states 7-9)
    A(7:9, 7:9) = [-2/3,  0,    0;
                     0,   -2/3,  0;
                     0,    0,   -2/3];
                     
    % RE Output Stage (states 10-13)
    A(10, 3:9) = [1, 0, 1, 0, 1, 1, 1];  % Connections from Solar and Wind
    A(10:13, 10:13) = [-1/4,  0,    0,    0;
                        0,   -1/4,   0,    0;
                        0,    0.6,   0,    0;
                        0,     0,    0,   -2];
                        
    % ESS (states 14-15)
    A(14:15, 14:15) = [-10,  0;
                         0, -10];
                         
    % Power System & Tie-lines (states 16-18)
    A(16, [1,10:15]) = [120/20, 120/20, 120/20, 120/20, 120/20, 120/20, 120/20];  % Effects on frequency
    A(16:18, 16:18) = [-1/20,  0,    0;
                        T12,    0,    0;  % Tie-line to MG1
                        T23,    0,    0];  % Tie-line to MG3
    
    % Input matrix B
    B = zeros(18, 1);
    B(1) = 1/2;  % Control input only affects DEG first state
    
    % Output matrix C - only measure frequency for control
    C = zeros(1, 18);
    C(16) = 1;  % Measure frequency state
    
    % Augmented System
    A_aug = [A, zeros(18,1);
             C, 0];
    B_aug = [B; 0];
    C_aug = [C, 0];
    
    % Discrete-time conversion
    Ad = eye(19) + Ts*A_aug;
    Bd = Ts*B_aug;
    Cd = C_aug;
    
    % Persistent variables with enhanced filtering
    persistent x_est u_prev integral_error avg_error filter_count
    persistent y_hist error_trend deltaPc_hist prev_solution
    persistent y_filtered_prev deltaPc_final_prev
    if isempty(x_est)
        x_est = zeros(19, 1);
        u_prev = 0;
        integral_error = 0;
        avg_error = 0;
        filter_count = 0;
        y_hist = zeros(8, 1);
        error_trend = zeros(5, 1);
        deltaPc_hist = zeros(3, 1);
        prev_solution = zeros(Nc, 1);
        y_filtered_prev = 0;
        deltaPc_final_prev = 0;
    end
    
    % Extract frequency information from neighbors
    freq_MG1 = neighbor_freqs(1);  % Leader frequency
    freq_MG3 = neighbor_freqs(2);
    
    % Distributed Control Based on Laplacian Matrix
    % For MG2 (Follower): Use neighboring information
    graph_gain = 0.2;  % Gain for graph-based control
    leader_gain = 0.5; % Higher gain for tracking the leader
    
    % Calculate distributed control error using graph theory
    % Based on local error + weighted neighbor errors
    laplacian_error = 2*local_freq - freq_MG1 - freq_MG3;
    leader_error = local_freq - freq_MG1;  % Track the leader
    
    % Combined error (follower node emphasizes tracking the leader)
    dist_error = leader_gain*leader_error + graph_gain*laplacian_error;
    
    % Enhanced measurement filtering with longer history and stronger filtering
    y_hist = [dist_error; y_hist(1:end-1)];
    
    % Two-stage filtering for maximum noise rejection
    % First stage: weighted moving average
    weights = [0.25, 0.2, 0.15, 0.1, 0.1, 0.08, 0.07, 0.05];
    weights = weights(1:min(length(weights), length(y_hist)));
    weights = weights / sum(weights);
    y_filtered_stage1 = y_hist' * weights';
    
    % Second stage: low-pass filter
    if isempty(y_filtered_prev)
        y_filtered_prev = y_filtered_stage1;
    end
    y_filtered = 0.8*y_filtered_prev + 0.2*y_filtered_stage1;
    y_filtered_prev = y_filtered;
    
    % Ultra-conservative integral action with wider dead zone
    error_signal = y_filtered;
    
    % Expanded dead zone with extremely slow integration
    if abs(error_signal) > 0.01
        integral_error = 0.99*integral_error + 0.01*Ts*error_signal*0.05;
    else
        % Inside dead zone - practically frozen integration
        integral_error = 0.9995*integral_error + 0.0005*Ts*error_signal*0.01;
    end
    
    % Moving average error for steady-state offset detection
    avg_error = 0.95*avg_error + 0.05*error_signal;
    filter_count = filter_count + 1;
    
    % State estimation with improved observer gain
    y_meas = y_filtered;
    x_est = Ad*x_est + Bd*u_prev;
    
    % Slightly increased observer gain for better tracking
    L = [0.08*ones(18,1); 0.12];
    x_est = x_est + L*(y_meas - Cd*x_est);
    x_est(19) = integral_error;
    
    % Prediction matrices
    [F, Phi] = getPredictionMatrices(Ad, Bd, Cd, Np, Nc);
    
    % Cost function weights - Critically over-damped response design
    % Extremely flat weight distribution for maximum smoothness
    %q_weights = exp(linspace(0, 0.2, Np));  % Very gradual weight increase
    Q = diag(500 * exp(linspace(0, 0.5, Np)));  % Sharper tracking
    
    % Ultra-high penalty on control moves to eliminate any oscillatory behavior
    R = diag(0.8 * ones(Nc,1));                 % Reduced control penalty
    
    % Reference trajectory - Targeting zero error
    r = zeros(Np,1);
    
    % Constraints - Extremely tight rate constraints for absolute stability
    du_max = 0.01;      % Minimal rate of change allowed
    u_max = 0.13;
    u_min = -0.13;
    
    % QP matrices
    [H, f] = getQPMatrices(F, Phi, Q, R, r, x_est);
    [A_ineq, b_ineq] = getConstraintMatrices(Nc, u_max, u_min, du_max, u_prev);
    
    % Initial guess - Use previous solution as starting point if available
    x0 = prev_solution;
    
    % Solve QP problem with improved options
    options = optimoptions('quadprog', 'Display', 'off', 'Algorithm', 'active-set', ...
                          'MaxIterations', 100);
    du = quadprog(H, f, A_ineq, b_ineq, [], [], [], [], x0, options);
    
    % Store solution for next iteration
    if ~isempty(du)
        prev_solution = du;
        delta_u = du(1);
    else
        delta_u = 0;
    end
    
    % Add anti-windup to prevent integral windup
    if abs(u_prev) >= u_max - 0.01
        integral_error = 0.9 * integral_error; % Reduce integral action when near constraints
    end
    
    % Maximum damping factor with triple-stage filtering
    % First stage - exponential smoothing with heavy bias toward previous value
    deltaPc_stage1 = 0.85*u_prev + 0.15*delta_u;
    
    % Second stage - moving average filter
    deltaPc_hist = [deltaPc_stage1; deltaPc_hist(1:end-1)];
    if all(deltaPc_hist == 0)
        deltaPc_hist = zeros(3, 1) + deltaPc_stage1;
    end
    deltaPc_stage2 = 0.7*deltaPc_hist(1) + 0.2*deltaPc_hist(2) + 0.1*deltaPc_hist(3);
    
    % Third stage - additional low-pass filter
    if isempty(deltaPc_final_prev)
        deltaPc_final_prev = deltaPc_stage2;
    end
    deltaPc = 0.9*deltaPc_final_prev + 0.1*deltaPc_stage2;
    deltaPc_final_prev = deltaPc;
    
    % Update persistent variables
    u_prev = deltaPc;
    
    return;
end

function [F, Phi] = getPredictionMatrices(A, B, C, Np, Nc)
    % Keep your existing function implementation
    [ny, nx] = size(C);
    F = zeros(Np, nx);
    Phi = zeros(Np, Nc);
    
    % Build F matrix
    for i = 1:Np
        F(i,:) = C * A^i;
    end
    
    % Build Phi matrix
    for i = 1:Np
        for j = 1:min(i,Nc)
            if i == j
                Phi(i,j) = C * B;
            else
                Phi(i,j) = C * A^(i-j) * B;
            end
        end
    end
end

function [H, f] = getQPMatrices(F, Phi, Q, R, r, x)
    % Keep your existing function implementation
    H = 2*(Phi'*Q*Phi + R);
    f = 2*Phi'*Q*(F*x - r);
end

function [A_ineq, b_ineq] = getConstraintMatrices(Nc, u_max, u_min, du_max, u_prev)
    % Keep your existing function implementation
    A_rate = [eye(Nc); -eye(Nc)];
    b_rate = [du_max*ones(Nc,1); du_max*ones(Nc,1)];
    
    A_input = tril(ones(Nc));
    A_amp = [A_input; -A_input];
    b_amp = [(u_max - u_prev)*ones(Nc,1); -(u_min - u_prev)*ones(Nc,1)];
    
    A_ineq = [A_rate; A_amp];
    b_ineq = [b_rate; b_amp];
end
